simulink model "SF020A_HwAgTrakgServo"  (R2013b)
settings: Solver=FixedStepDiscrete  SolverMode=SingleTasking  StartTime=0.0  StopTime=1  FixedStep=0.002  RelTol=1e-3
undefined symbols (not defined in the file): ARCHGLBPRM_2MILLISEC_SEC_F32, HwAgTrakgServoEnaRate, HwAgTrakgServoExecRate, HwAgTrakgServoMaxRamp, HwAgTrakgServoPidLim, HwAgTrakgServoRampCmpl, SYSGLBPRM_MOTTQCMDHILIM_MOTNWTMTR_F32, SYSGLBPRM_MOTTQCMDLOLIM_MOTNWTMTR_F32
libraries: FixdToFloat x9, FloatToFixd x8, LnrIntrpn x7, NxtrLim x7, Fil x6, simulink x3, NxtrAbslt x2, BilnrIntrpnCmnX x2, NxtrSign x2
(part 1 of 2)
settings Model: Creator=VZBTJX  LastModifiedBy=VZBTJX
settings SolverCC: AutoInsertRateTranBlk=on  InsertRTBMode=Always
settings DataIOCC: LimitDataPoints=off  SaveFormat=Structure  ReturnWorkspaceOutputs=on
settings OptimizationCC: BlockReduction=off  InlineParams=on  ZeroExternalMemoryAtStartup=off  ZeroInternalMemoryAtStartup=off  OptimizeModelRefInitCode=on  LifeSpan=1
settings DebuggingCC: SignalInfNanChecking=error  SignalRangeChecking=warning  ReadBeforeWriteMsg=EnableAllAsWarning  WriteAfterWriteMsg=EnableAllAsWarning  WriteAfterReadMsg=EnableAllAsWarning  UnderspecifiedInitializationDetection=Simplified  SolverPrmCheckMsg=error  InheritedTsInSrcMsg=error  DiscreteInheritContinuousMsg=error  SingleTaskRateTransMsg=error  TasksWithSamePriorityMsg=error  SigSpecEnsureSampleTimeMsg=error  CheckMatrixSingularityMsg=error  ParameterUnderflowMsg=error  ParameterPrecisionLossMsg=error  ParameterTunabilityLossMsg=error  FixptConstUnderflowMsg=warning  FixptConstOverflowMsg=warning  VectorMatrixConversionMsg=error  SignalLabelMismatchMsg=error  UnconnectedInputMsg=error  UnconnectedOutputMsg=error  UnconnectedLineMsg=error  SFcnCompatibilityMsg=error  UniqueDataStoreMsg=warning  BusObjectLabelMismatch=error  RootOutportRequireBusObject=error  AssertControl=DisableAll  ModelReferenceIOMsg=error  ModelReferenceVersionMismatchMessage=warning  ModelReferenceIOMismatchMessage=error  ModelReferenceCSMismatchMessage=warning  ModelReferenceDataLoggingMessage=error  StateNameClashWarn=warning  StrictBusMsg=ErrorOnBusTreatedAsVector  NonBusSignalsTreatedAsBus=error  SFUnexpectedBacktrackingDiag=error  SFInvalidInputDataAccessInChartInitDiag=error  SFNoUnconditionalDefaultTransitionDiag=error  SFTransitionOutsideNaturalParentDiag=error  SFUnconditionalTransitionShadowingDiag=error  SFUndirectedBroadcastEventsDiag=error
settings ModelReferenceCC: ModelReferenceNumInstancesAllowed=Single
settings RTWCC: SystemTargetFile=autosar.tlc  GenCodeOnly=on  TemplateMakefile=ert_default_tmf  Description=AUTOSAR  GenerateReport=on  ProcessScript=autosar_make_rtw_hook  LaunchReport=on
settings CodeAppCC: GenerateComments=off  IgnoreCustomStorageClasses=off  CustomSymbolStrType=$N$R$M  CustomSymbolStrBlkIO=$N$M  SimulinkBlockComments=off
settings STFCustomTargetCC: ParMdlRefBuildCompliant=on  CompOptLevelCompliant=on  IncludeMdlTerminateFcn=off  CombineOutputUpdateFcns=on  SuppressErrorStatus=on  ERTFirstTimeCompliant=on  ERTCustomFileBanners=on  SupportNonFinite=off  SupportComplex=off  SupportContinuousTime=off  SupportNonInlinedSFcns=off  MATLABClassNameForMDSCustomization=Simulink.SoftwareTarget.ERTCustomization  AutosarCompliant=on  GRTInterface=off  SystemTargetFile=autosar.tlc
settings ERTTargetCC: CodeReplacementLibrary=ANSI_C  ConcurrentExecutionCompliant=off  IncludeMdlTerminateFcn=off  SuppressErrorStatus=on  SupportNonFinite=off  SupportComplex=off  ModelStepFunctionPrototypeControlCompliant=off  CPPClassGenCompliant=off  AutosarCompliant=on  InlinedParameterPlacement=NonHierarchical  ERTCustomFileTemplate=example_file_process.tlc  EnableUserReplacementTypes=on

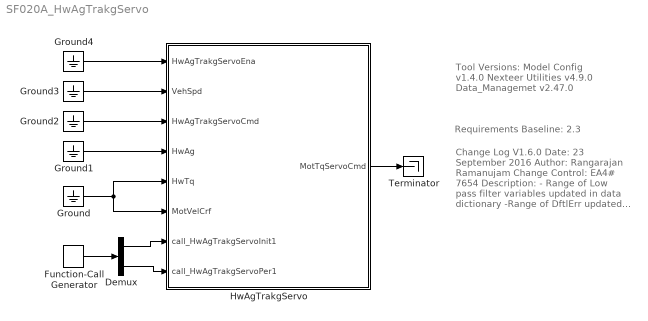
== system SF020A_HwAgTrakgServo ==
  note: Requirements Baseline: 2.3
  note: Tool Versions:
      |
      | Model Config v1.4.0
      | Nexteer Utilities v4.9.0
      | Data_Managemet v2.47.0
  note: Change Log
      |
      | V1.6.0
      | Date: 23 September 2016
      | Author: Rangarajan Ramanujam
      | Change Control: EA4# 7654
      | Description:
      | - Range of Low pass filter variables updated
      | in data dictionary
      | -Range of DftlErr updated in data dictionary
      |
      | V1.5.0
      | - Range of PrevIntglErr updated in
      | the data dictionary.
      | - Removed gain block in the subsystem
      | 'D-Term'.
      |
      | V1.4.0
      | Date: 17 Aug 2016
      | Author :Rangarajan Ramanujam
      | Change control : EA4#6955
      | Description:
      | - Vehicle Speed converstion from
      | u8p8 to u9p7 in DD and model
      | - Absolute HwAgErr lookup
      | changed from u10p6 to u12p4 to
      | in DD and model
      |
      | V1.3.0
      | - Updated the datatype of Cal
      | 'HwAgTrakgServoDampgTq'
      | to u11p5 in DD and model.
      |
      | V1.2.2
      | Author :Rangarajan Ramanujam
      | Description:
      | -ASIL Safety rating corrected in
      | requirements
      |
      | V1.2.1
      | Author :Rangarajan Ramanujam
      | Description:
      | -Requirements traced to Model
      |
      | V1.2.0
      | Author :Rangarajan Ramanujam
      | Description:
      | -Model corrections to accomodate
      | allowable comparisons of signals
      |
      | V1.1.0
      | Author :Rangarajan Ramanujam
      | Description:
      | -Corrections made to model to
      | match data types
      |
      | V1.0.0
      | Author :Rangarajan Ramanujam
      | Description:
      | - Initial Release
      | - Based on V005 of EA3
      | - Level 1 Model
  Demux : Demux  Outputs=2
  Function-Call Generator : simulink/Ports & Subsystems/Function-Call Generator  sample_time=1  numberOfIterations=1
  Ground{,1..4} (5 alike) : Ground
  HwAgTrakgServo : Subsystem
  Terminator : Terminator
  wires:
  HwAgTrakgServo/1(MotTqServoCmd) -> Terminator/1
  Function-Call Generator/1 -> Demux/1
  Demux/1 -> HwAgTrakgServo/7(call_HwAgTrakgServoInit1)
  Demux/2 -> HwAgTrakgServo/8(call_HwAgTrakgServoPer1)
  Ground/1 -> HwAgTrakgServo/6(MotVelCrf), HwAgTrakgServo/5(HwTq)
  Ground4/1 -> HwAgTrakgServo/1(HwAgTrakgServoEna)
  Ground3/1 -> HwAgTrakgServo/2(VehSpd)
  Ground2/1 -> HwAgTrakgServo/3(HwAgTrakgServoCmd)
  Ground1/1 -> HwAgTrakgServo/4(HwAg)

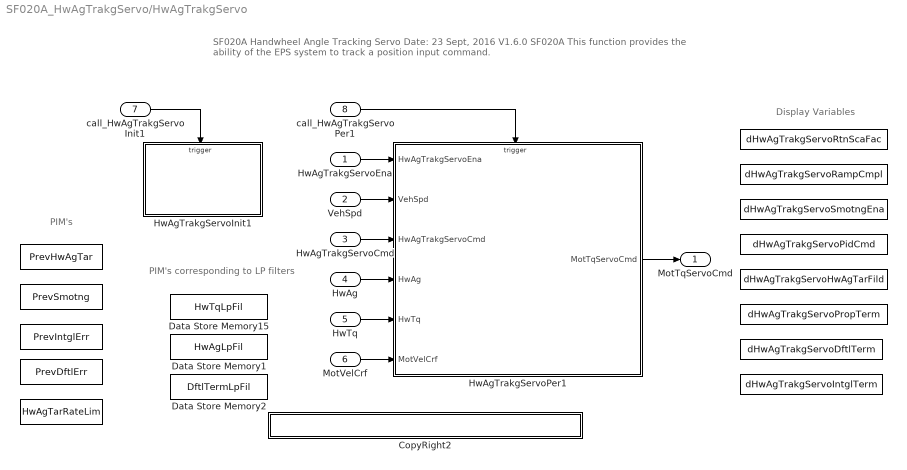
== system SF020A_HwAgTrakgServo/HwAgTrakgServo ==
  note: PIM's
  note: Display Variables
  note: PIM's corresponding to LP filters
  note: SF020A  Handwheel Angle Tracking Servo					Date:  23 Sept, 2016
      | V1.6.0
      |
      | SF020A
      | This function provides the ability of the EPS system to track a position input command.
  HwAgTrakgServoEna : Inport  RequirementInfo={'linktype_rmi_doors' '0000a533 (/E-STEER Core/SubSystem Specifications/Application Functions/SF020A Position Tracking Servo)' '#SF020A_9' 'true' 'REQ:SF020A_9' '' } %GIDa_0a861a63_eae7_41df_a6b9_e4ac69c247c6
  VehSpd : Inport  RequirementInfo={'linktype_rmi_doors' '0000a533 (/E-STEER Core/SubSystem Specifications/Application Functions/SF020A Position Tracking Servo)' '#SF020A_32' 'true' 'REQ:SF020A_32' '' } %GIDa_9975bceb_7073_4ae0_b4dc_116f23096c75  Port=2
  HwAgTrakgServoCmd : Inport  RequirementInfo={'linktype_rmi_doors' '0000a533 (/E-STEER Core/SubSystem Specifications/Application Functions/SF020A Position Tracking Servo)' '#SF020A_33' 'true' 'REQ:SF020A_33' '' } %GIDa_a09b565d_8dea_44d0_8fa8_fd4ac32c0e32  Port=3
  HwAg : Inport  RequirementInfo={'linktype_rmi_doors' '0000a533 (/E-STEER Core/SubSystem Specifications/Application Functions/SF020A Position Tracking Servo)' '#SF020A_34' 'true' 'REQ:SF020A_34' '' } %GIDa_ee6dde83_a75d_439c_9d63_2038ff9dde1a  Port=4
  HwTq : Inport  RequirementInfo={'linktype_rmi_doors' '0000a533 (/E-STEER Core/SubSystem Specifications/Application Functions/SF020A Position Tracking Servo)' '#SF020A_35' 'true' 'REQ:SF020A_35' '' } %GIDa_76a33000_2421_4445_bb2d_c6af0fdfcce8  Port=5
  MotVelCrf : Inport  RequirementInfo={'linktype_rmi_doors' '0000a533 (/E-STEER Core/SubSystem Specifications/Application Functions/SF020A Position Tracking Servo)' '#SF020A_36' 'true' 'REQ:SF020A_36' '' } %GIDa_8ec51612_5d38_4e63_91bd_22aea72136a4  Port=6
  call_HwAgTrakgServoInit1 : Inport  Port=7
  call_HwAgTrakgServoPer1 : Inport  Port=8
  " " : DataStoreMemory  DataStoreName=dHwAgTrakgServoRtnScaFac  ReadBeforeWriteMsg=warning  WriteAfterWriteMsg=warning  WriteAfterReadMsg=warning  InitialValue=[]  StateMustResolveToSignalObject=on
  "  " : DataStoreMemory  DataStoreName=dHwAgTrakgServoPidCmd  ReadBeforeWriteMsg=warning  WriteAfterWriteMsg=warning  WriteAfterReadMsg=warning  InitialValue=[]  StateMustResolveToSignalObject=on
  "   " : DataStoreMemory  DataStoreName=dHwAgTrakgServoSmotngEna  ReadBeforeWriteMsg=warning  WriteAfterWriteMsg=warning  WriteAfterReadMsg=warning  InitialValue=[]  StateMustResolveToSignalObject=on
  " " : DataStoreMemory  DataStoreName=dHwAgTrakgServoPropTerm  ReadBeforeWriteMsg=warning  WriteAfterWriteMsg=warning  WriteAfterReadMsg=warning  InitialValue=[]  StateMustResolveToSignalObject=on
  "     " : DataStoreMemory  DataStoreName=dHwAgTrakgServoRampCmpl  ReadBeforeWriteMsg=warning  WriteAfterWriteMsg=warning  WriteAfterReadMsg=warning  InitialValue=[]  StateMustResolveToSignalObject=on
  "         " : DataStoreMemory  DataStoreName=PrevHwAgTar  ReadBeforeWriteMsg=warning  WriteAfterWriteMsg=warning  WriteAfterReadMsg=warning  StateMustResolveToSignalObject=on
  " " : DataStoreMemory  DataStoreName=dHwAgTrakgServoDftlTerm  ReadBeforeWriteMsg=warning  WriteAfterWriteMsg=warning  WriteAfterReadMsg=warning  InitialValue=[]  StateMustResolveToSignalObject=on
  " " : DataStoreMemory  DataStoreName=dHwAgTrakgServoIntglTerm  ReadBeforeWriteMsg=warning  WriteAfterWriteMsg=warning  WriteAfterReadMsg=warning  InitialValue=[]  StateMustResolveToSignalObject=on
  " " : DataStoreMemory  DataStoreName=PrevIntglErr  ReadBeforeWriteMsg=warning  WriteAfterWriteMsg=warning  WriteAfterReadMsg=warning  StateMustResolveToSignalObject=on
  "                  " : DataStoreMemory  DataStoreName=dHwAgTrakgServoHwAgTarFild  ReadBeforeWriteMsg=warning  WriteAfterWriteMsg=warning  WriteAfterReadMsg=warning  InitialValue=[]  StateMustResolveToSignalObject=on
  "                                         " : DataStoreMemory  DataStoreName=PrevSmotng  ReadBeforeWriteMsg=warning  WriteAfterWriteMsg=warning  WriteAfterReadMsg=warning  StateMustResolveToSignalObject=on
  "                                                                        " : DataStoreMemory  DataStoreName=HwAgTarRateLim  ReadBeforeWriteMsg=warning  WriteAfterWriteMsg=warning  WriteAfterReadMsg=warning  StateMustResolveToSignalObject=on
  "                                                                            " : DataStoreMemory  DataStoreName=PrevDftlErr  ReadBeforeWriteMsg=warning  WriteAfterWriteMsg=warning  WriteAfterReadMsg=warning  StateMustResolveToSignalObject=on
  CopyRight2 : Subsystem  Description=|  mask(Copyright Information){none=on}
      | Copyright info block.                                               
      |                                                                     
      | Place copyright information at the top of every subsystem in design.
      mask prompts: none "No parameters"
      mask help: Place copyright information at the top of every subsystem in design.
      mask Display:
      | NxtrConf = 'Nexteer Confidential';
      | 
      | sys = bdroot; %handle for the current model ("system")
      | first = get_param(sys,'Created');
      | first = first(end-3:end);  %year is last four digits
      | 
      | last = get_param(sys,'LastModifiedDate');
      | if isempty(last)
      |     last = datestr(now,'yyyy');
      | else
      |     last = last(end-3:end);
      | end
      | 
      | if strcmp(first,last)
      |     fprintf('%s -- Copyright %s Nexteer',NxtrConf,first)
      | else
      |     fprintf('%s -- %s%s- %s Nexteer',NxtrConf,char(169),first,last)
      | end
  Data Store Memory1 : DataStoreMemory  DataStoreName=HwAgLpFil  InitialValue=[]  OutDataTypeStr=Bus: FilLpRec1  StateMustResolveToSignalObject=on
  Data Store Memory15 : DataStoreMemory  DataStoreName=HwTqLpFil  InitialValue=[]  OutDataTypeStr=Bus: FilLpRec1  StateMustResolveToSignalObject=on
  Data Store Memory2 : DataStoreMemory  DataStoreName=DftlTermLpFil  InitialValue=[]  OutDataTypeStr=Bus: FilLpRec1  StateMustResolveToSignalObject=on
  HwAgTrakgServoInit1 : Subsystem
  HwAgTrakgServoPer1 : Subsystem
  MotTqServoCmd : Outport  RequirementInfo={'linktype_rmi_doors' '0000a533 (/E-STEER Core/SubSystem Specifications/Application Functions/SF020A Position Tracking Servo)' '#SF020A_11' 'true' 'REQ:SF020A_11' '' } %GIDa_fe7a3d0d_243b_4dee_aede_3d564675bb1a
  wires:
  HwAgTrakgServoEna/1 -> HwAgTrakgServoPer1/1(HwAgTrakgServoEna)
  VehSpd/1 -> HwAgTrakgServoPer1/2(VehSpd)
  HwAgTrakgServoCmd/1 -> HwAgTrakgServoPer1/3(HwAgTrakgServoCmd)
  HwAg/1 -> HwAgTrakgServoPer1/4(HwAg)
  HwTq/1 -> HwAgTrakgServoPer1/5(HwTq)
  MotVelCrf/1 -> HwAgTrakgServoPer1/6(MotVelCrf)
  HwAgTrakgServoPer1/1(MotTqServoCmd) -> MotTqServoCmd/1
  call_HwAgTrakgServoInit1/1 -> HwAgTrakgServoInit1/Trigger
  call_HwAgTrakgServoPer1/1 -> HwAgTrakgServoPer1/Trigger

== system SF020A_HwAgTrakgServo/HwAgTrakgServo/CopyRight2 ==

== system SF020A_HwAgTrakgServo/HwAgTrakgServo/HwAgTrakgServoInit1 ==
  function : TriggerPort  TriggerType=function-call
  CopyRight2 : Subsystem  Description=|  mask(Copyright Information){none=on}
      | Copyright info block.                                               
      |                                                                     
      | Place copyright information at the top of every subsystem in design.
      mask prompts: none "No parameters"
      mask help: Place copyright information at the top of every subsystem in design.
      mask Display:
      | NxtrConf = 'Nexteer Confidential';
      | 
      | sys = bdroot; %handle for the current model ("system")
      | first = get_param(sys,'Created');
      | if(isempty(first))
      |     first = datestr(now,'yyyy');
      | else
      |     first = first(end-3:end);  %year is last four digits
      | end
      | 
      | last = get_param(sys,'LastModifiedDate');
      | if isempty(last)
      |     last = datestr(now,'yyyy');
      | else
      |     last = last(end-3:end);
      | end
      | 
      | if strcmp(first,last)
      |     fprintf('%s -- Copyright %s Nexteer',NxtrConf,first)
      | else
      |     fprintf('%s -- %s%s- %s Nexteer',NxtrConf,char(169),first,last)
      | end
  DftlTermLpFil : Fil/FilLpInit  Ic=0  Ts=ARCHGLBPRM_2MILLISEC_SEC_F32  Freq=HwAgTrakgServoDftlTermLpFilFrq  StVar=DftlTermLpFil
  HwAgLpFil : Fil/FilLpInit  Ic=0  Ts=ARCHGLBPRM_2MILLISEC_SEC_F32  Freq=HwAgTrakgServoHwAgLpFilFrq  StVar=HwAgLpFil
  HwTqLpFil : Fil/FilLpInit  Ic=0  Ts=ARCHGLBPRM_2MILLISEC_SEC_F32  Freq=HwAgTrakgServoHwTqLpFilFrq  StVar=HwTqLpFil

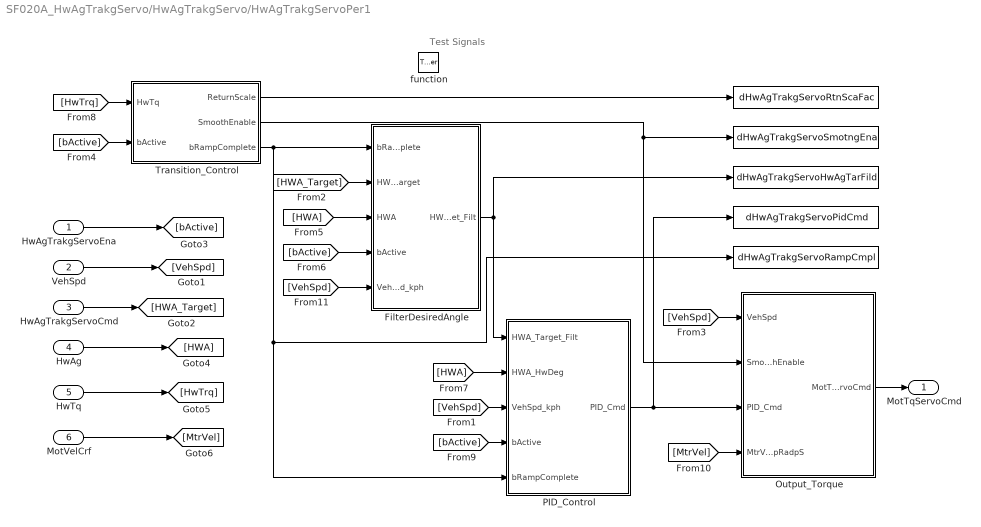
== system SF020A_HwAgTrakgServo/HwAgTrakgServo/HwAgTrakgServoPer1 ==
  note: Test Signals
  HwAgTrakgServoEna : Inport
  VehSpd : Inport  Port=2
  HwAgTrakgServoCmd : Inport  Port=3
  HwAg : Inport  Port=4
  HwTq : Inport  Port=5
  MotVelCrf : Inport  Port=6
  function : TriggerPort  TriggerType=function-call
  "       " : DataStoreWrite  DataStoreName=dHwAgTrakgServoRtnScaFac
  " " : DataStoreWrite  DataStoreName=dHwAgTrakgServoPidCmd
  " " : DataStoreWrite  DataStoreName=dHwAgTrakgServoSmotngEna
  "                          " : DataStoreWrite  DataStoreName=dHwAgTrakgServoRampCmpl
  " " : DataStoreWrite  DataStoreName=dHwAgTrakgServoHwAgTarFild
  FilterDesiredAngle : Subsystem
  Output_Torque : Subsystem
  PID_Control : Subsystem
  Transition_Control : Subsystem
  MotTqServoCmd : Outport
  wires:
  Transition_Control/1(ReturnScale) -> "       "/1
  Output_Torque/1(MotTqServoCmd) -> MotTqServoCmd/1
  Transition_Control/3(bRampComplete) -> FilterDesiredAngle/1(bRampComplete), PID_Control/5(bRampComplete), "                          "/1
  FilterDesiredAngle/1(HWA_Target_Filt) -> " "/1, PID_Control/1(HWA_Target_Filt)
  [bActive] -> FilterDesiredAngle/4(bActive)
  [HWA] -> FilterDesiredAngle/3(HWA)
  [HWA_Target] -> FilterDesiredAngle/2(HWA_Target)
  [MtrVel] -> Output_Torque/4(MtrVel_MtrNmpRadpS)
  [bActive] -> PID_Control/4(bActive)
  [VehSpd] -> PID_Control/3(VehSpd_kph)
  [HWA] -> PID_Control/2(HWA_HwDeg)
  [bActive] -> Transition_Control/2(bActive)
  [HwTrq] -> Transition_Control/1(HwTq)
  Transition_Control/2(SmoothEnable) -> Output_Torque/2(SmoothEnable), " "/1
  [VehSpd] -> Output_Torque/1(VehSpd)
  PID_Control/1(PID_Cmd) -> " "/1, Output_Torque/3(PID_Cmd)
  MotVelCrf/1 -> [MtrVel]
  HwAgTrakgServoEna/1 -> [bActive]
  VehSpd/1 -> [VehSpd]
  HwAgTrakgServoCmd/1 -> [HWA_Target]
  HwAg/1 -> [HWA]
  HwTq/1 -> [HwTrq]
  [VehSpd] -> FilterDesiredAngle/5(VehSpd_kph)

== system SF020A_HwAgTrakgServo/HwAgTrakgServo/HwAgTrakgServoInit1/CopyRight2 ==

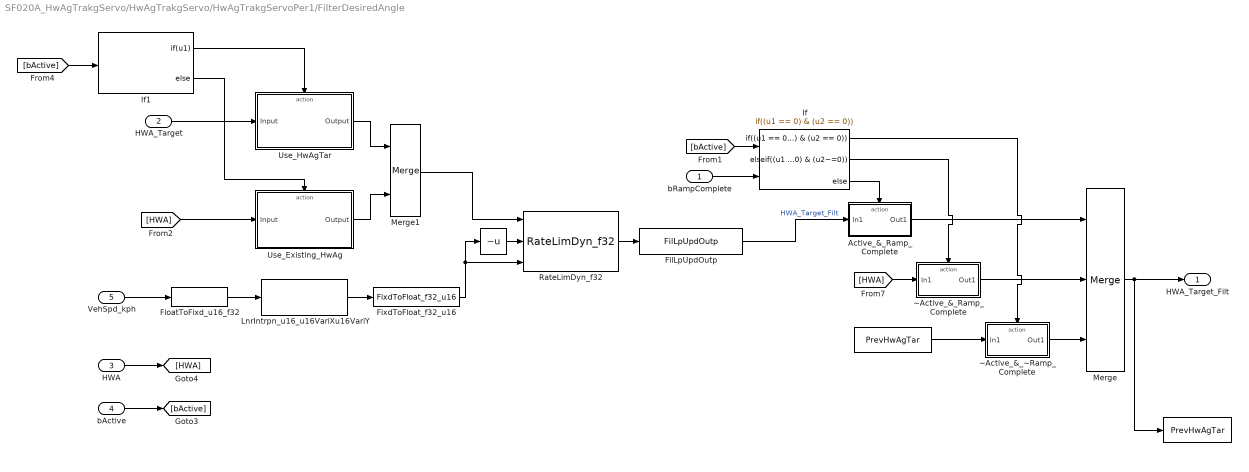
== system SF020A_HwAgTrakgServo/HwAgTrakgServo/HwAgTrakgServoPer1/FilterDesiredAngle ==
  bRampComplete : Inport
  HWA_Target : Inport  RequirementInfo={'linktype_rmi_doors' '0000a533 (/E-STEER Core/SubSystem Specifications/Application Functions/SF020A Position Tracking Servo)' '#SF020A_99' 'true' 'REQ:SF020A_99' '' } %GIDa_e7acc575_0f73_464f_afbf_a1d3f2ef75c3  Port=2
  HWA : Inport  Port=3
  bActive : Inport  Port=4
  VehSpd_kph : Inport  RequirementInfo={'linktype_rmi_doors' '0000a533 (/E-STEER Core/SubSystem Specifications/Application Functions/SF020A Position Tracking Servo)' '#SF020A_99' 'true' 'REQ:SF020A_99' '' } %GIDa_85b9ae16_376e_449a_90e2_5040a7306451  Port=5
  " " : UnaryMinus  RequirementInfo={'linktype_rmi_doors' '0000a533 (/E-STEER Core/SubSystem Specifications/Application Functions/SF020A Position Tracking Servo)' '#SF020A_99' 'true' 'REQ:SF020A_99' '' } %GIDa_efd44ab5_c18e_4f6b_b334_c09a99d942d0
  "     " : DataStoreWrite  DataStoreName=PrevHwAgTar
  "        " : DataStoreRead  RequirementInfo={'linktype_rmi_doors' '0000a533 (/E-STEER Core/SubSystem Specifications/Application Functions/SF020A Position Tracking Servo)' '#SF020A_101' 'true' 'REQ:SF020A_101' '' } %GIDa_6c1952a9_0ffa_4be9_8189_fa3e3336d45c  DataStoreName=PrevHwAgTar
  Active_&_Ramp_Complete : Subsystem  RequirementInfo={'linktype_rmi_doors' '0000a533 (/E-STEER Core/SubSystem Specifications/Application Functions/SF020A Position Tracking Servo)' '#SF020A_99' 'true' 'REQ:SF020A_99' '' } %GIDa_4a952202_34bf_43ef_8f0f_aa433087b1b9  TreatAsAtomicUnit=on
  FilLpUpdOutp : Fil/FilLpUpdOutp  RequirementInfo="{'linktype_rmi_doors' '0000a533 (/E-STEER Core/SubSystem Specifications/Application Functions/SF020A Position Tracking Servo)' '#SF020A_99' 'true' 'REQ:  SF020A_99' '' } %GIDa_b3db9956_e025_4d49_9afa_1bbba3a9e619"  StVar=HwAgLpFil
      settings: AttributesFormatString=StVar: %<StVar>
  FixdToFloat_f32_u16 : FixdToFloat/FixdToFloat_f32_u16  RequirementInfo="{'linktype_rmi_doors' '0000a533 (/E-STEER Core/SubSystem Specifications/Application Functions/SF020A Position Tracking Servo)' '#SF020A_99' 'true' 'REQ:  SF020A_99' '' } %GIDa_c0d72d1d_c5d3_483f_995f_11228bcef0f6"  Param1=6
  FloatToFixd_u16_f32 : FloatToFixd/FloatToFixd_u16_f32  RequirementInfo="{'linktype_rmi_doors' '0000a533 (/E-STEER Core/SubSystem Specifications/Application Functions/SF020A Position Tracking Servo)' '#SF020A_99' 'true' 'REQ:  SF020A_99' '' } %GIDa_9b4afccd_8bf2_4923_94b9_643f59fca2d5"  Param1=7
  If : If  NumInputs=2  IfExpression=(u1 == 0) & (u2 == 0)  ElseIfExpressions=(u1 ==0) & (u2~=0)
  If1 : If  RequirementInfo={} %GIDa_a4efa7cf_020b_4e2c_8b39_ca1fe09c08dd  IfExpression=u1
  LnrIntrpn_u16_u16VariXu16VariY : LnrIntrpn/LnrIntrpn_u16_u16VariXu16VariY  RequirementInfo="{'linktype_rmi_doors' '0000a533 (/E-STEER Core/SubSystem Specifications/Application Functions/SF020A Position Tracking Servo)' '#SF020A_99' 'true' 'REQ:  SF020A_99' '' } %GIDa_8d1c4332_48e0_4b17_889c_946355c87589"  XTbl=HwAgTrakgServoVehSpdBasd  YTbl=HwAgTrakgServoHwAgRateLim
      settings: AttributesFormatString=Lnr ( u16VariX , u16VariY )
  Merge : Merge  Inputs=3
  Merge1 : Merge
  RateLimDyn_f32 : NxtrLim/RateLimDyn_f32  RequirementInfo="{'linktype_rmi_doors' '0000a533 (/E-STEER Core/SubSystem Specifications/Application Functions/SF020A Position Tracking Servo)' '#SF020A_99' 'true' 'REQ:  SF020A_99' '' } %GIDa_e8b1a6d3_31e8_44b3_82da_7d89fe70b03c"  StVar=HwAgTarRateLim  Ts=ARCHGLBPRM_2MILLISEC_SEC_F32
      settings: AttributesFormatString=StVar: %<StVar>
  Use_Existing_HwAg : Subsystem  RequirementInfo={} %GIDa_50f4cb49_8adf_449a_b42e_90dc65779533  TreatAsAtomicUnit=on
  Use_HwAgTar : Subsystem  RequirementInfo={'linktype_rmi_doors' '0000a533 (/E-STEER Core/SubSystem Specifications/Application Functions/SF020A Position Tracking Servo)' '#SF020A_99' 'true' 'REQ:SF020A_99' '' } %GIDa_668d9e3b_eeaa_4a0b_876a_e6d874a9d4ce  TreatAsAtomicUnit=on
  ~Active_&_Ramp_Complete : Subsystem  RequirementInfo={'linktype_rmi_doors' '0000a533 (/E-STEER Core/SubSystem Specifications/Application Functions/SF020A Position Tracking Servo)' '#SF020A_100' 'true' 'REQ:SF020A_100' '' } %GIDa_817091e4_3589_4307_8098_766d3e0f9054  TreatAsAtomicUnit=on
  ~Active_&_~Ramp_Complete : Subsystem  RequirementInfo={'linktype_rmi_doors' '0000a533 (/E-STEER Core/SubSystem Specifications/Application Functions/SF020A Position Tracking Servo)' '#SF020A_101' 'true' 'REQ:SF020A_101' '' } %GIDa_b19d96da_ebcd_4204_9ab1_e486e7ddf7b1  TreatAsAtomicUnit=on
  HWA_Target_Filt : Outport  RequirementInfo={'linktype_rmi_doors' '0000a533 (/E-STEER Core/SubSystem Specifications/Application Functions/SF020A Position Tracking Servo)' '#SF020A_98' 'true' 'REQ:SF020A_98' '' } %GIDa_868abe07_be0e_45ba_867f_1ff711be68fc
  wires:
  [bActive] -> If/1
  bRampComplete/1 -> If/2
  If/3 -> Active_&_Ramp_Complete/Action
  If/2 -> ~Active_&_Ramp_Complete/Action
  If/1 -> ~Active_&_~Ramp_Complete/Action
  Active_&_Ramp_Complete/1(Out1) -> Merge/1
  ~Active_&_Ramp_Complete/1(Out1) -> Merge/2
  ~Active_&_~Ramp_Complete/1(Out1) -> Merge/3
  Merge/1 -> "     "/1, HWA_Target_Filt/1
  FilLpUpdOutp/1 -> Active_&_Ramp_Complete/1(In1)  "HWA_Target_Filt"
  [HWA] -> ~Active_&_Ramp_Complete/1(In1)
  VehSpd_kph/1 -> FloatToFixd_u16_f32/1
  RateLimDyn_f32/1 -> FilLpUpdOutp/1
  FixdToFloat_f32_u16/1 -> " "/1, RateLimDyn_f32/3
  " "/1 -> RateLimDyn_f32/2
  HWA/1 -> [HWA]
  bActive/1 -> [bActive]
  FloatToFixd_u16_f32/1 -> LnrIntrpn_u16_u16VariXu16VariY/1
  LnrIntrpn_u16_u16VariXu16VariY/1 -> FixdToFloat_f32_u16/1
  If1/1 -> Use_HwAgTar/Action
  If1/2 -> Use_Existing_HwAg/Action
  [bActive] -> If1/1
  HWA_Target/1 -> Use_HwAgTar/1(Input)
  Merge1/1 -> RateLimDyn_f32/1
  Use_Existing_HwAg/1(Output) -> Merge1/2
  Use_HwAgTar/1(Output) -> Merge1/1
  "        "/1 -> ~Active_&_~Ramp_Complete/1(In1)
  [HWA] -> Use_Existing_HwAg/1(Input)

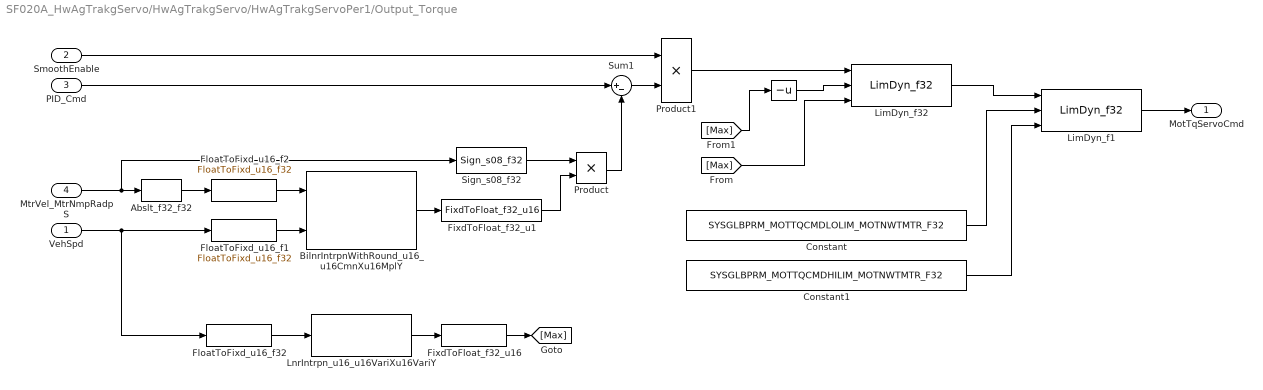
== system SF020A_HwAgTrakgServo/HwAgTrakgServo/HwAgTrakgServoPer1/Output_Torque ==
  VehSpd : Inport  RequirementInfo={'linktype_rmi_doors' '0000a533 (/E-STEER Core/SubSystem Specifications/Application Functions/SF020A Position Tracking Servo)' '#SF020A_127' 'true' 'REQ:SF020A_127' '' } %GIDa_474620a4_325b_4492_8ecd_3526588549a0
  SmoothEnable : Inport  RequirementInfo={'linktype_rmi_doors' '0000a533 (/E-STEER Core/SubSystem Specifications/Application Functions/SF020A Position Tracking Servo)' '#SF020A_127' 'true' 'REQ:SF020A_127' '' } %GIDa_9a858461_1c5b_449a_a972_5d559b949f50  Port=2
  PID_Cmd : Inport  RequirementInfo={'linktype_rmi_doors' '0000a533 (/E-STEER Core/SubSystem Specifications/Application Functions/SF020A Position Tracking Servo)' '#SF020A_127' 'true' 'REQ:SF020A_127' '' } %GIDa_052b79db_c29f_4d5a_af97_6b714f3815b4  Port=3
  MtrVel_MtrNmpRadpS : Inport  RequirementInfo={'linktype_rmi_doors' '0000a533 (/E-STEER Core/SubSystem Specifications/Application Functions/SF020A Position Tracking Servo)' '#SF020A_127' 'true' 'REQ:SF020A_127' '' } %GIDa_1f627eb9_1ad5_4c89_915a_5692511d3e0e  Port=4
  "  " : UnaryMinus  RequirementInfo={'linktype_rmi_doors' '0000a533 (/E-STEER Core/SubSystem Specifications/Application Functions/SF020A Position Tracking Servo)' '#SF020A_128' 'true' 'REQ:SF020A_128' '' } %GIDa_208b4a7f_e90f_4a28_aeb5_84bf42b1973c
  Abslt_f32_f32 : NxtrAbslt/Abslt_f32_f32  RequirementInfo="{'linktype_rmi_doors' '0000a533 (/E-STEER Core/SubSystem Specifications/Application Functions/SF020A Position Tracking Servo)' '#SF020A_127' 'true' 'REQ:  SF020A_127' '' } %GIDa_4c7f84e2_9c51_4ac4_bc8e_368a17407767"  SFunctionSpec=single y1 = Abslt_f32_f32(single u1)
      settings: AttributesFormatString=%<Name>
  BilnrIntrpnWithRound_u16_u16CmnXu16MplY : BilnrIntrpnCmnX/BilnrIntrpnWithRound_u16_u16CmnXu16MplY  RequirementInfo="{'linktype_rmi_doors' '0000a533 (/E-STEER Core/SubSystem Specifications/Application Functions/SF020A Position Tracking Servo)' '#SF020A_127' 'true' 'REQ:  SF020A_127' '' } %GIDa_c34291a5_3911_408b_8b47_f05b2755e6cc"  XTbl=HwAgTrakgServoDampgTqX  MplYTbl=HwAgTrakgServoDampgTqY  BilnrSelnTbl=HwAgTrakgServoVehSpdBasd
      settings: AttributesFormatString=Bilnr ( u16CmnX , u16MplY )
  Constant : Constant  Value=SYSGLBPRM_MOTTQCMDLOLIM_MOTNWTMTR_F32
  Constant1 : Constant  Value=SYSGLBPRM_MOTTQCMDHILIM_MOTNWTMTR_F32
  FixdToFloat_f32_u1 : FixdToFloat/FixdToFloat_f32_u16  RequirementInfo="{'linktype_rmi_doors' '0000a533 (/E-STEER Core/SubSystem Specifications/Application Functions/SF020A Position Tracking Servo)' '#SF020A_127' 'true' 'REQ:  SF020A_127' '' } %GIDa_87bb9503_9691_42e0_a96a_59d3106357c3"  Param1=12
  FixdToFloat_f32_u16 : FixdToFloat/FixdToFloat_f32_u16  RequirementInfo="{'linktype_rmi_doors' '0000a533 (/E-STEER Core/SubSystem Specifications/Application Functions/SF020A Position Tracking Servo)' '#SF020A_128' 'true' 'REQ:  SF020A_128' '' } %GIDa_5017700d_fcd6_4af6_9979_9b8b09242964"  Param1=12
  FloatToFixd_u16_f1 : FloatToFixd/FloatToFixd_u16_f32  RequirementInfo="{'linktype_rmi_doors' '0000a533 (/E-STEER Core/SubSystem Specifications/Application Functions/SF020A Position Tracking Servo)' '#SF020A_127' 'true' 'REQ:  SF020A_127' '' } %GIDa_c2c61aee_7eb3_4b4a_87cd_5695f0b08806"  Param1=7
  FloatToFixd_u16_f2 : FloatToFixd/FloatToFixd_u16_f32  RequirementInfo="{'linktype_rmi_doors' '0000a533 (/E-STEER Core/SubSystem Specifications/Application Functions/SF020A Position Tracking Servo)' '#SF020A_127' 'true' 'REQ:  SF020A_127' '' } %GIDa_803faa1d_8b83_4ad8_ac94_947faa679a05"  Param1=5
  FloatToFixd_u16_f32 : FloatToFixd/FloatToFixd_u16_f32  RequirementInfo="{'linktype_rmi_doors' '0000a533 (/E-STEER Core/SubSystem Specifications/Application Functions/SF020A Position Tracking Servo)' '#SF020A_128' 'true' 'REQ:  SF020A_128' '' } %GIDa_aa6e0d64_6b9c_4ee5_97e1_061e01469387"  Param1=7
  LimDyn_f1 : NxtrLim/LimDyn_f32
  LimDyn_f32 : NxtrLim/LimDyn_f32  RequirementInfo="{'linktype_rmi_doors' '0000a533 (/E-STEER Core/SubSystem Specifications/Application Functions/SF020A Position Tracking Servo)' '#SF020A_128' 'true' 'REQ:  SF020A_128' '' } %GIDa_c1077bf5_3047_48c9_a12c_9eeda7f5db36"
  LnrIntrpn_u16_u16VariXu16VariY : LnrIntrpn/LnrIntrpn_u16_u16VariXu16VariY  RequirementInfo="{'linktype_rmi_doors' '0000a533 (/E-STEER Core/SubSystem Specifications/Application Functions/SF020A Position Tracking Servo)' '#SF020A_128' 'true' 'REQ:  SF020A_128' '' } %GIDa_1fa861a0_a179_48d3_a99b_f33a8b13458b"  XTbl=HwAgTrakgServoMaxCmdX  YTbl=HwAgTrakgServoMaxCmdY
      settings: AttributesFormatString=Lnr ( u16VariX , u16VariY )
  Product : Product  RequirementInfo={'linktype_rmi_doors' '0000a533 (/E-STEER Core/SubSystem Specifications/Application Functions/SF020A Position Tracking Servo)' '#SF020A_127' 'true' 'REQ:SF020A_127' '' } %GIDa_4fb66050_b8f6_4af8_96e6_10fec13bb5b1  RndMeth=Zero
  Product1 : Product  RequirementInfo={'linktype_rmi_doors' '0000a533 (/E-STEER Core/SubSystem Specifications/Application Functions/SF020A Position Tracking Servo)' '#SF020A_127' 'true' 'REQ:SF020A_127' '' } %GIDa_c01da8b7_40de_4569_a775_6186fd8f6704  RndMeth=Zero
  Sign_s08_f32 : NxtrSign/Sign_s08_f32  RequirementInfo="{'linktype_rmi_doors' '0000a533 (/E-STEER Core/SubSystem Specifications/Application Functions/SF020A Position Tracking Servo)' '#SF020A_127' 'true' 'REQ:  SF020A_127' '' } %GIDa_8db97c32_7333_4b68_8940_025c4fe6d06f"  SFunctionSpec=int8 y1 = Sign_s08_f32(single u1)
  Sum1 : Sum  RequirementInfo={'linktype_rmi_doors' '0000a533 (/E-STEER Core/SubSystem Specifications/Application Functions/SF020A Position Tracking Servo)' '#SF020A_127' 'true' 'REQ:SF020A_127' '' } %GIDa_0169afd4_386e_427c_bfd4_53921aeb59b7  Inputs=|+-
  MotTqServoCmd : Outport  RequirementInfo={'linktype_rmi_doors' '0000a533 (/E-STEER Core/SubSystem Specifications/Application Functions/SF020A Position Tracking Servo)' '#SF020A_126' 'true' 'REQ:SF020A_126' '' } %GIDa_f5d4f1fd_008c_428f_b74f_f026ee59aaf7
  wires:
  MtrVel_MtrNmpRadpS/1 -> Sign_s08_f32/1, Abslt_f32_f32/1
  FixdToFloat_f32_u1/1 -> Product/2
  Sum1/1 -> Product1/2
  Product1/1 -> LimDyn_f32/1
  SmoothEnable/1 -> Product1/1
  PID_Cmd/1 -> Sum1/1
  VehSpd/1 -> FloatToFixd_u16_f32/1, FloatToFixd_u16_f1/1
  "  "/1 -> LimDyn_f32/2
  FixdToFloat_f32_u16/1 -> [Max]
  [Max] -> LimDyn_f32/3
  [Max] -> "  "/1
  Sign_s08_f32/1 -> Product/1
  Product/1 -> Sum1/2
  FloatToFixd_u16_f1/1 -> BilnrIntrpnWithRound_u16_u16CmnXu16MplY/2
  FloatToFixd_u16_f2/1 -> BilnrIntrpnWithRound_u16_u16CmnXu16MplY/1
  BilnrIntrpnWithRound_u16_u16CmnXu16MplY/1 -> FixdToFloat_f32_u1/1
  Abslt_f32_f32/1 -> FloatToFixd_u16_f2/1
  FloatToFixd_u16_f32/1 -> LnrIntrpn_u16_u16VariXu16VariY/1
  LnrIntrpn_u16_u16VariXu16VariY/1 -> FixdToFloat_f32_u16/1
  LimDyn_f1/1 -> MotTqServoCmd/1
  LimDyn_f32/1 -> LimDyn_f1/1
  Constant/1 -> LimDyn_f1/2
  Constant1/1 -> LimDyn_f1/3

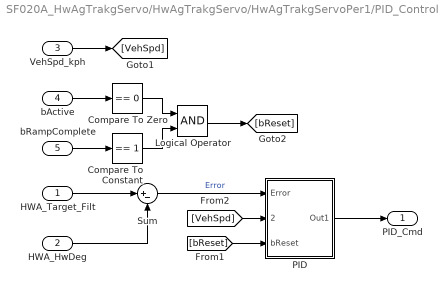
== system SF020A_HwAgTrakgServo/HwAgTrakgServo/HwAgTrakgServoPer1/PID_Control ==
  HWA_Target_Filt : Inport  RequirementInfo={'linktype_rmi_doors' '0000a533 (/E-STEER Core/SubSystem Specifications/Application Functions/SF020A Position Tracking Servo)' '#SF020A_102' 'true' 'REQ:SF020A_102' '' } %GIDa_96554c5e_998d_4f15_83f9_911c59ccdd83
  HWA_HwDeg : Inport  RequirementInfo={'linktype_rmi_doors' '0000a533 (/E-STEER Core/SubSystem Specifications/Application Functions/SF020A Position Tracking Servo)' '#SF020A_102' 'true' 'REQ:SF020A_102' '' } %GIDa_6ee0171f_9720_4863_a2bf_ea00195cf774  Port=2
  VehSpd_kph : Inport  Port=3
  bActive : Inport  RequirementInfo={'linktype_rmi_doors' '0000a533 (/E-STEER Core/SubSystem Specifications/Application Functions/SF020A Position Tracking Servo)' '#SF020A_103' 'true' 'REQ:SF020A_103' '' } %GIDa_9eddb9e0_5e8f_4f17_9b84_ed84197a6fc3  Port=4
  bRampComplete : Inport  RequirementInfo={'linktype_rmi_doors' '0000a533 (/E-STEER Core/SubSystem Specifications/Application Functions/SF020A Position Tracking Servo)' '#SF020A_103' 'true' 'REQ:SF020A_103' '' } %GIDa_355cbabc_0398_4c34_81ee_416f63569dc9  Port=5
  Compare To Constant : simulink/Logic and Bit Operations/Compare To Constant  RequirementInfo="{'linktype_rmi_doors' '0000a533 (/E-STEER Core/SubSystem Specifications/Application Functions/SF020A Position Tracking Servo)' '#SF020A_103' 'true' 'REQ:  SF020A_103' '' } %GIDa_2eb7b152_7ccc_4248_9fc6_46fce54e4617"  relop===  const=1  OutDataTypeStr=boolean  ZeroCross=off
  Compare To Zero : simulink/Logic and Bit Operations/Compare To Zero  RequirementInfo="{'linktype_rmi_doors' '0000a533 (/E-STEER Core/SubSystem Specifications/Application Functions/SF020A Position Tracking Servo)' '#SF020A_103' 'true' 'REQ:  SF020A_103' '' } %GIDa_6b434ffe_ee5c_4534_8f75_3b9fed22d920"  relop===  OutDataTypeStr=boolean  ZeroCross=off
  Logical Operator : Logic  RequirementInfo={'linktype_rmi_doors' '0000a533 (/E-STEER Core/SubSystem Specifications/Application Functions/SF020A Position Tracking Servo)' '#SF020A_103' 'true' 'REQ:SF020A_103' '' } %GIDa_f2747463_b12c_42b8_b260_d601006f7267  AllPortsSameDT=off  OutDataTypeStr=boolean
  PID : Subsystem
  Sum : Sum  RequirementInfo={'linktype_rmi_doors' '0000a533 (/E-STEER Core/SubSystem Specifications/Application Functions/SF020A Position Tracking Servo)' '#SF020A_102' 'true' 'REQ:SF020A_102' '' } %GIDa_8c1b8298_9b52_4497_850d_13288e77f55f  Inputs=|+-
  PID_Cmd : Outport
  wires:
  HWA_Target_Filt/1 -> Sum/1
  HWA_HwDeg/1 -> Sum/2
  Sum/1 -> PID/1(Error)  "Error"
  VehSpd_kph/1 -> [VehSpd]
  bActive/1 -> Compare To Zero/1
  [bReset] -> PID/3(bReset)
  [VehSpd] -> PID/2(VehSpd)
  PID/1(Out1) -> PID_Cmd/1
  bRampComplete/1 -> Compare To Constant/1
  Compare To Zero/1 -> Logical Operator/1
  Compare To Constant/1 -> Logical Operator/2
  Logical Operator/1 -> [bReset]

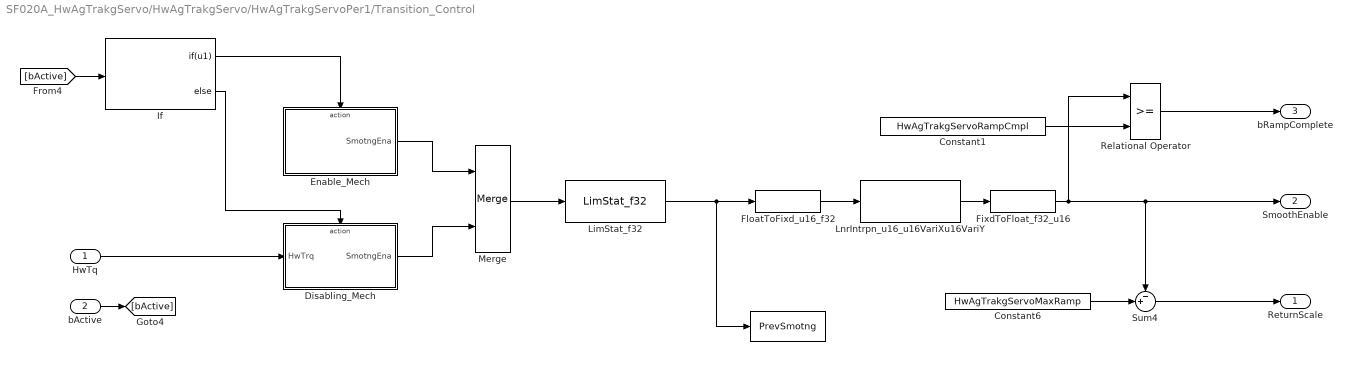
== system SF020A_HwAgTrakgServo/HwAgTrakgServo/HwAgTrakgServoPer1/Transition_Control ==
  HwTq : Inport
  bActive : Inport  Port=2
  "     " : DataStoreWrite  DataStoreName=PrevSmotng
  Constant1 : Constant  RequirementInfo={'linktype_rmi_doors' '0000a533 (/E-STEER Core/SubSystem Specifications/Application Functions/SF020A Position Tracking Servo)' '#SF020A_95' 'true' 'REQ:SF020A_95' '' ; 'linktype_rmi_doors' '0000a533 (/E-STEER Core/SubSystem Specifications/Application Functions/SF020A Position Tracking Servo)' '#SF020A_96' 'true' 'REQ:SF020A_96' '' } %GIDa_cb099e48_7da0_468e_a3b0_a4077127fdf5  Value=HwAgTrakgServoRampCmpl
  Constant6 : Constant  Value=HwAgTrakgServoMaxRamp
  Disabling_Mech : Subsystem  RequirementInfo={} %GIDa_f3aa73c0_63ab_4d72_b303_f53c42d5dfe3  TreatAsAtomicUnit=on
  Enable_Mech : Subsystem  RequirementInfo={} %GIDa_038a4bb2_1fce_4620_8407_5e4359fcd734  TreatAsAtomicUnit=on
  FixdToFloat_f32_u16 : FixdToFloat/FixdToFloat_f32_u16  RequirementInfo="{'linktype_rmi_doors' '0000a533 (/E-STEER Core/SubSystem Specifications/Application Functions/SF020A Position Tracking Servo)' '#SF020A_70' 'true' 'REQ:  SF020A_70' '' } %GIDa_a82123da_8349_4491_b0dc_e6121eefd7a1"  Param1=15
  FloatToFixd_u16_f32 : FloatToFixd/FloatToFixd_u16_f32  RequirementInfo="{'linktype_rmi_doors' '0000a533 (/E-STEER Core/SubSystem Specifications/Application Functions/SF020A Position Tracking Servo)' '#SF020A_70' 'true' 'REQ:  SF020A_70' '' } %GIDa_2eacbca8_6954_4120_9199_a15501379883"  Param1=15
  If : If  RequirementInfo={} %GIDa_c593b6c1_44d8_4555_b2bc_14652956d79f  IfExpression=u1
  LimStat_f32 : NxtrLim/LimStat_f32  RequirementInfo="{'linktype_rmi_doors' '0000a533 (/E-STEER Core/SubSystem Specifications/Application Functions/SF020A Position Tracking Servo)' '#SF020A_70' 'true' 'REQ:  SF020A_70' '' } %GIDa_4fb8fd50_52bf_48b4_95a4_8b1359686cec"  LoLim=HwAgTrakgServoMinRamp  HiLim=HwAgTrakgServoMaxRamp
      settings: AttributesFormatString=|
      | Low Limit: %<LoLim>
      | High Limit:%<HiLim>
  LnrIntrpn_u16_u16VariXu16VariY : LnrIntrpn/LnrIntrpn_u16_u16VariXu16VariY  RequirementInfo="{'linktype_rmi_doors' '0000a533 (/E-STEER Core/SubSystem Specifications/Application Functions/SF020A Position Tracking Servo)' '#SF020A_70' 'true' 'REQ:  SF020A_70' '' } %GIDa_869739a1_3e56_4785_b0b9_37fd25a35bb8"  XTbl=HwAgTrakgServoSmotngX  YTbl=HwAgTrakgServoSmotngY
      settings: AttributesFormatString=Lnr ( u16VariX , u16VariY )
  Merge : Merge
  Relational Operator : RelationalOperator  RequirementInfo={'linktype_rmi_doors' '0000a533 (/E-STEER Core/SubSystem Specifications/Application Functions/SF020A Position Tracking Servo)' '#SF020A_95' 'true' 'REQ:SF020A_95' '' ; 'linktype_rmi_doors' '0000a533 (/E-STEER Core/SubSystem Specifications/Application Functions/SF020A Position Tracking Servo)' '#SF020A_96' 'true' 'REQ:SF020A_96' '' } %GIDa_12123dec_37ee_44a5_86a0_f897b93fae09  OutDataTypeStr=boolean
  Sum4 : Sum  Inputs=-+|
  ReturnScale : Outport
  SmoothEnable : Outport  RequirementInfo={'linktype_rmi_doors' '0000a533 (/E-STEER Core/SubSystem Specifications/Application Functions/SF020A Position Tracking Servo)' '#SF020A_69' 'true' 'REQ:SF020A_69' '' } %GIDa_5e249da6_f5f8_4dc6_9c6b_71bc17b083ab  Port=2
  bRampComplete : Outport  RequirementInfo={'linktype_rmi_doors' '0000a533 (/E-STEER Core/SubSystem Specifications/Application Functions/SF020A Position Tracking Servo)' '#SF020A_94' 'true' 'REQ:SF020A_94' '' } %GIDa_da62325a_8fb5_4022_854a_4674025e36d9  Port=3
  wires:
  Constant6/1 -> Sum4/2
  FixdToFloat_f32_u16/1 -> Relational Operator/1, Sum4/1, SmoothEnable/1
  LimStat_f32/1 -> "     "/1, FloatToFixd_u16_f32/1
  Merge/1 -> LimStat_f32/1
  Sum4/1 -> ReturnScale/1
  bActive/1 -> [bActive]
  Constant1/1 -> Relational Operator/2
  Relational Operator/1 -> bRampComplete/1
  HwTq/1 -> Disabling_Mech/1(HwTrq)
  [bActive] -> If/1
  If/1 -> Enable_Mech/Action
  Enable_Mech/1(SmotngEna) -> Merge/1
  If/2 -> Disabling_Mech/Action
  Disabling_Mech/1(SmotngEna) -> Merge/2
  FloatToFixd_u16_f32/1 -> LnrIntrpn_u16_u16VariXu16VariY/1
  LnrIntrpn_u16_u16VariXu16VariY/1 -> FixdToFloat_f32_u16/1

== system SF020A_HwAgTrakgServo/HwAgTrakgServo/HwAgTrakgServoPer1/FilterDesiredAngle/Active_&_Ramp_Complete ==
  In1 : Inport
  Action Port : ActionPort  ActionType=else
  Out1 : Outport
  wires:
  In1/1 -> Out1/1

== system SF020A_HwAgTrakgServo/HwAgTrakgServo/HwAgTrakgServoPer1/FilterDesiredAngle/Use_Existing_HwAg ==
  Input : Inport
  Action Port : ActionPort  ActionType=else
  CopyRight2 : Subsystem  Description=|  mask(Copyright Information){none=on}
      | Copyright info block.                                               
      |                                                                     
      | Place copyright information at the top of every subsystem in design.
      mask prompts: none "No parameters"
      mask help: Place copyright information at the top of every subsystem in design.
      mask Display:
      | NxtrConf = 'Nexteer Confidential';
      | 
      | sys = bdroot; %handle for the current model ("system")
      | first = get_param(sys,'Created');
      | if(isempty(first))
      |     first = datestr(now,'yyyy');
      | else
      |     first = first(end-3:end);  %year is last four digits
      | end
      | 
      | last = get_param(sys,'LastModifiedDate');
      | if isempty(last)
      |     last = datestr(now,'yyyy');
      | else
      |     last = last(end-3:end);
      | end
      | 
      | if strcmp(first,last)
      |     fprintf('%s -- Copyright %s Nexteer',NxtrConf,first)
      | else
      |     fprintf('%s -- %s%s- %s Nexteer',NxtrConf,char(169),first,last)
      | end
  Output : Outport
  wires:
  Input/1 -> Output/1

== system SF020A_HwAgTrakgServo/HwAgTrakgServo/HwAgTrakgServoPer1/FilterDesiredAngle/Use_HwAgTar ==
  Input : Inport
  Action Port : ActionPort  ActionType=then
  CopyRight2 : Subsystem  Description=|  mask(Copyright Information){none=on}
      | Copyright info block.                                               
      |                                                                     
      | Place copyright information at the top of every subsystem in design.
      mask prompts: none "No parameters"
      mask help: Place copyright information at the top of every subsystem in design.
      mask Display:
      | NxtrConf = 'Nexteer Confidential';
      | 
      | sys = bdroot; %handle for the current model ("system")
      | first = get_param(sys,'Created');
      | if(isempty(first))
      |     first = datestr(now,'yyyy');
      | else
      |     first = first(end-3:end);  %year is last four digits
      | end
      | 
      | last = get_param(sys,'LastModifiedDate');
      | if isempty(last)
      |     last = datestr(now,'yyyy');
      | else
      |     last = last(end-3:end);
      | end
      | 
      | if strcmp(first,last)
      |     fprintf('%s -- Copyright %s Nexteer',NxtrConf,first)
      | else
      |     fprintf('%s -- %s%s- %s Nexteer',NxtrConf,char(169),first,last)
      | end
  Output : Outport
  wires:
  Input/1 -> Output/1

== system SF020A_HwAgTrakgServo/HwAgTrakgServo/HwAgTrakgServoPer1/FilterDesiredAngle/~Active_&_Ramp_Complete ==
  In1 : Inport
  Action Port : ActionPort  ActionType=elseif
  Out1 : Outport
  wires:
  In1/1 -> Out1/1

== system SF020A_HwAgTrakgServo/HwAgTrakgServo/HwAgTrakgServoPer1/FilterDesiredAngle/~Active_&_~Ramp_Complete ==
  In1 : Inport
  Action Port : ActionPort  ActionType=then
  Out1 : Outport
  wires:
  In1/1 -> Out1/1

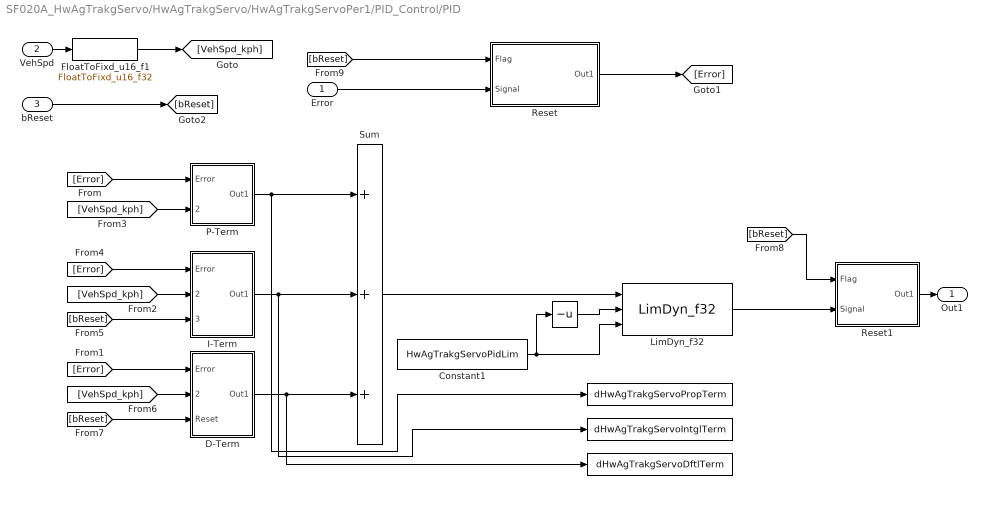
== system SF020A_HwAgTrakgServo/HwAgTrakgServo/HwAgTrakgServoPer1/PID_Control/PID ==
  Error : Inport  RequirementInfo={'linktype_rmi_doors' '0000a533 (/E-STEER Core/SubSystem Specifications/Application Functions/SF020A Position Tracking Servo)' '#SF020A_104' 'true' 'REQ:SF020A_104' '' } %GIDa_f15145c7_6000_4779_b1f7_48eb6fb6ad1e
  VehSpd : Inport  Port=2
  bReset : Inport  Port=3
  " " : UnaryMinus  RequirementInfo={'linktype_rmi_doors' '0000a533 (/E-STEER Core/SubSystem Specifications/Application Functions/SF020A Position Tracking Servo)' '#SF020A_124' 'true' 'REQ:SF020A_124' '' } %GIDa_a76ad962_7874_4290_b490_84c06de5e485
  "                          " : DataStoreWrite  DataStoreName=dHwAgTrakgServoPropTerm
  "                            " : DataStoreWrite  DataStoreName=dHwAgTrakgServoIntglTerm
  "                                   " : DataStoreWrite  DataStoreName=dHwAgTrakgServoDftlTerm
  Constant1 : Constant  RequirementInfo={'linktype_rmi_doors' '0000a533 (/E-STEER Core/SubSystem Specifications/Application Functions/SF020A Position Tracking Servo)' '#SF020A_124' 'true' 'REQ:SF020A_124' '' } %GIDa_0069e4e2_8656_446c_bf95_2f4427c8e623  Value=HwAgTrakgServoPidLim
  D-Term : Subsystem
  FloatToFixd_u16_f1 : FloatToFixd/FloatToFixd_u16_f32  Param1=7
  I-Term : Subsystem
  LimDyn_f32 : NxtrLim/LimDyn_f32  RequirementInfo="{'linktype_rmi_doors' '0000a533 (/E-STEER Core/SubSystem Specifications/Application Functions/SF020A Position Tracking Servo)' '#SF020A_124' 'true' 'REQ:  SF020A_124' '' } %GIDa_57432fac_f525_482c_b2ff_f7dc1f9d906b"
  P-Term : Subsystem
  Reset : Subsystem  RequirementInfo={'linktype_rmi_doors' '0000a533 (/E-STEER Core/SubSystem Specifications/Application Functions/SF020A Position Tracking Servo)' '#SF020A_104' 'true' 'REQ:SF020A_104' '' } %GIDa_f659e05c_2c1f_4734_852d_fbd34a2b0812
  Reset1 : Subsystem  RequirementInfo={'linktype_rmi_doors' '0000a533 (/E-STEER Core/SubSystem Specifications/Application Functions/SF020A Position Tracking Servo)' '#SF020A_125' 'true' 'REQ:SF020A_125' '' } %GIDa_701216af_0a80_491e_95b0_6581edba11ae
  Sum : Sum  RequirementInfo={'linktype_rmi_doors' '0000a533 (/E-STEER Core/SubSystem Specifications/Application Functions/SF020A Position Tracking Servo)' '#SF020A_123' 'true' 'REQ:SF020A_123' '' } %GIDa_ec60f3e8_bd63_4182_9416_2c9793cf7f05  Inputs=+++
  Out1 : Outport
  wires:
  Error/1 -> Reset/2(Signal)
  VehSpd/1 -> FloatToFixd_u16_f1/1
  [Error] -> P-Term/1(Error)
  [VehSpd_kph] -> P-Term/2(VehSpd)
  [Error] -> I-Term/1(Error)
  [VehSpd_kph] -> I-Term/2(VehSpd)
  bReset/1 -> [bReset]
  [bReset] -> I-Term/3(bReset)
  Sum/1 -> LimDyn_f32/1
  [Error] -> D-Term/1(Error)
  [VehSpd_kph] -> D-Term/2(VehSpd)
  P-Term/1(Out1) -> "                          "/1, Sum/1
  I-Term/1(Out1) -> "                            "/1, Sum/2
  D-Term/1(Out1) -> "                                   "/1, Sum/3
  [bReset] -> D-Term/3(Reset)
  [bReset] -> Reset1/1(Flag)
  Reset1/1(Out1) -> Out1/1
  [bReset] -> Reset/1(Flag)
  Reset/1(Out1) -> [Error]
  LimDyn_f32/1 -> Reset1/2(Signal)
  FloatToFixd_u16_f1/1 -> [VehSpd_kph]
  Constant1/1 -> LimDyn_f32/3, " "/1
  " "/1 -> LimDyn_f32/2

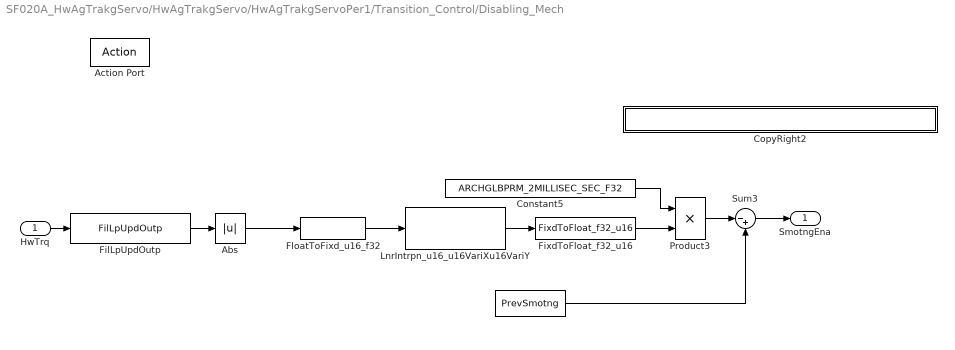
== system SF020A_HwAgTrakgServo/HwAgTrakgServo/HwAgTrakgServoPer1/Transition_Control/Disabling_Mech ==
  HwTrq : Inport
  Action Port : ActionPort  ActionType=else
  " " : DataStoreRead  RequirementInfo={'linktype_rmi_doors' '0000a533 (/E-STEER Core/SubSystem Specifications/Application Functions/SF020A Position Tracking Servo)' '#SF020A_93' 'true' 'REQ:SF020A_93' '' } %GIDa_0b9ad58e_3b3a_4fd4_ba45_d7e5a45f84ce  DataStoreName=PrevSmotng
  Abs : Abs  RequirementInfo={'linktype_rmi_doors' '0000a533 (/E-STEER Core/SubSystem Specifications/Application Functions/SF020A Position Tracking Servo)' '#SF020A_93' 'true' 'REQ:SF020A_93' '' } %GIDa_8389354a_cc04_49e8_832c_ef62a0072520
  Constant5 : Constant  RequirementInfo={'linktype_rmi_doors' '0000a533 (/E-STEER Core/SubSystem Specifications/Application Functions/SF020A Position Tracking Servo)' '#SF020A_93' 'true' 'REQ:SF020A_93' '' } %GIDa_174158a4_9368_4900_9431_fd4fb8c48a59  Value=ARCHGLBPRM_2MILLISEC_SEC_F32
  CopyRight2 : Subsystem  Description=|  mask(Copyright Information){none=on}
      | Copyright info block.                                               
      |                                                                     
      | Place copyright information at the top of every subsystem in design.
      mask prompts: none "No parameters"
      mask help: Place copyright information at the top of every subsystem in design.
      mask Display:
      | NxtrConf = 'Nexteer Confidential';
      | 
      | sys = bdroot; %handle for the current model ("system")
      | first = get_param(sys,'Created');
      | if(isempty(first))
      |     first = datestr(now,'yyyy');
      | else
      |     first = first(end-3:end);  %year is last four digits
      | end
      | 
      | last = get_param(sys,'LastModifiedDate');
      | if isempty(last)
      |     last = datestr(now,'yyyy');
      | else
      |     last = last(end-3:end);
      | end
      | 
      | if strcmp(first,last)
      |     fprintf('%s -- Copyright %s Nexteer',NxtrConf,first)
      | else
      |     fprintf('%s -- %s%s- %s Nexteer',NxtrConf,char(169),first,last)
      | end
  FilLpUpdOutp : Fil/FilLpUpdOutp  RequirementInfo="{'linktype_rmi_doors' '0000a533 (/E-STEER Core/SubSystem Specifications/Application Functions/SF020A Position Tracking Servo)' '#SF020A_93' 'true' 'REQ:  SF020A_93' '' } %GIDa_31abe3b9_1629_4f64_99be_e505146e9c64"  StVar=HwTqLpFil
      settings: AttributesFormatString=StVar: %<StVar>
  FixdToFloat_f32_u16 : FixdToFloat/FixdToFloat_f32_u16  RequirementInfo="{'linktype_rmi_doors' '0000a533 (/E-STEER Core/SubSystem Specifications/Application Functions/SF020A Position Tracking Servo)' '#SF020A_93' 'true' 'REQ:  SF020A_93' '' } %GIDa_1402f738_529a_406f_88b3_9559060dea3d"  Param1=9
  FloatToFixd_u16_f32 : FloatToFixd/FloatToFixd_u16_f32  RequirementInfo="{'linktype_rmi_doors' '0000a533 (/E-STEER Core/SubSystem Specifications/Application Functions/SF020A Position Tracking Servo)' '#SF020A_93' 'true' 'REQ:  SF020A_93' '' } %GIDa_2d523958_94c1_4087_ab88_d132a6d98aa2"  Param1=12
  LnrIntrpn_u16_u16VariXu16VariY : LnrIntrpn/LnrIntrpn_u16_u16VariXu16VariY  RequirementInfo="{'linktype_rmi_doors' '0000a533 (/E-STEER Core/SubSystem Specifications/Application Functions/SF020A Position Tracking Servo)' '#SF020A_93' 'true' 'REQ:  SF020A_93' '' } %GIDa_abfd248b_35f4_4d51_a50a_76719713b517"  XTbl=HwAgTrakgServoDiRateX  YTbl=HwAgTrakgServoDiRateY
      settings: AttributesFormatString=Lnr ( u16VariX , u16VariY )
  Product3 : Product  RequirementInfo={'linktype_rmi_doors' '0000a533 (/E-STEER Core/SubSystem Specifications/Application Functions/SF020A Position Tracking Servo)' '#SF020A_93' 'true' 'REQ:SF020A_93' '' } %GIDa_09246e54_ae41_4398_b0ad_c319f8b255e4  RndMeth=Zero
  Sum3 : Sum  RequirementInfo={'linktype_rmi_doors' '0000a533 (/E-STEER Core/SubSystem Specifications/Application Functions/SF020A Position Tracking Servo)' '#SF020A_93' 'true' 'REQ:SF020A_93' '' } %GIDa_ada5bc2b_821a_4aa1_a182_296f7ff89c57  Inputs=|-+
  SmotngEna : Outport  InitialOutput=[0]
  wires:
  Product3/1 -> Sum3/1
  Abs/1 -> FloatToFixd_u16_f32/1
  FixdToFloat_f32_u16/1 -> Product3/2
  Constant5/1 -> Product3/1
  FilLpUpdOutp/1 -> Abs/1
  HwTrq/1 -> FilLpUpdOutp/1
  FloatToFixd_u16_f32/1 -> LnrIntrpn_u16_u16VariXu16VariY/1
  LnrIntrpn_u16_u16VariXu16VariY/1 -> FixdToFloat_f32_u16/1
  Sum3/1 -> SmotngEna/1
  " "/1 -> Sum3/2

== system SF020A_HwAgTrakgServo/HwAgTrakgServo/HwAgTrakgServoPer1/Transition_Control/Enable_Mech ==
  Action Port : ActionPort  ActionType=then
  " " : DataStoreRead  RequirementInfo={'linktype_rmi_doors' '0000a533 (/E-STEER Core/SubSystem Specifications/Application Functions/SF020A Position Tracking Servo)' '#SF020A_71' 'true' 'REQ:SF020A_71' '' } %GIDa_2760107c_b68f_40c1_abaa_5bba7198126a  DataStoreName=PrevSmotng
  Constant3 : Constant  RequirementInfo={'linktype_rmi_doors' '0000a533 (/E-STEER Core/SubSystem Specifications/Application Functions/SF020A Position Tracking Servo)' '#SF020A_71' 'true' 'REQ:SF020A_71' '' } %GIDa_e39f339b_849e_43c5_b02a_27a38bd6c821  Value=ARCHGLBPRM_2MILLISEC_SEC_F32
  Constant4 : Constant  RequirementInfo={'linktype_rmi_doors' '0000a533 (/E-STEER Core/SubSystem Specifications/Application Functions/SF020A Position Tracking Servo)' '#SF020A_71' 'true' 'REQ:SF020A_71' '' } %GIDa_fcf3289c_4e50_423f_91fe_51ee7e94c6fd  Value=HwAgTrakgServoEnaRate
  CopyRight2 : Subsystem  Description=|  mask(Copyright Information){none=on}
      | Copyright info block.                                               
      |                                                                     
      | Place copyright information at the top of every subsystem in design.
      mask prompts: none "No parameters"
      mask help: Place copyright information at the top of every subsystem in design.
      mask Display:
      | NxtrConf = 'Nexteer Confidential';
      | 
      | sys = bdroot; %handle for the current model ("system")
      | first = get_param(sys,'Created');
      | if(isempty(first))
      |     first = datestr(now,'yyyy');
      | else
      |     first = first(end-3:end);  %year is last four digits
      | end
      | 
      | last = get_param(sys,'LastModifiedDate');
      | if isempty(last)
      |     last = datestr(now,'yyyy');
      | else
      |     last = last(end-3:end);
      | end
      | 
      | if strcmp(first,last)
      |     fprintf('%s -- Copyright %s Nexteer',NxtrConf,first)
      | else
      |     fprintf('%s -- %s%s- %s Nexteer',NxtrConf,char(169),first,last)
      | end
  Product2 : Product  RequirementInfo={'linktype_rmi_doors' '0000a533 (/E-STEER Core/SubSystem Specifications/Application Functions/SF020A Position Tracking Servo)' '#SF020A_71' 'true' 'REQ:SF020A_71' '' } %GIDa_52c5c206_7c61_424f_8540_ff12a5ebfc0e  RndMeth=Zero
  Sum2 : Sum  RequirementInfo={'linktype_rmi_doors' '0000a533 (/E-STEER Core/SubSystem Specifications/Application Functions/SF020A Position Tracking Servo)' '#SF020A_71' 'true' 'REQ:SF020A_71' '' } %GIDa_1b259fe6_e371_495e_af54_7838b303cf47  Inputs=++|
  SmotngEna : Outport  RequirementInfo={'linktype_rmi_doors' '0000a533 (/E-STEER Core/SubSystem Specifications/Application Functions/SF020A Position Tracking Servo)' '#SF020A_71' 'true' 'REQ:SF020A_71' '' } %GIDa_a1b88202_ffa4_446e_a996_654e0d945e2d  InitialOutput=[0]
  wires:
  Sum2/1 -> SmotngEna/1
  Product2/1 -> Sum2/2
  Constant4/1 -> Product2/2
  Constant3/1 -> Product2/1
  " "/1 -> Sum2/1

== system SF020A_HwAgTrakgServo/HwAgTrakgServo/HwAgTrakgServoPer1/FilterDesiredAngle/Use_Existing_HwAg/CopyRight2 ==

== system SF020A_HwAgTrakgServo/HwAgTrakgServo/HwAgTrakgServoPer1/FilterDesiredAngle/Use_HwAgTar/CopyRight2 ==
